simulink model "Electrical_System_2018b_obfs"  (R2019b)
settings: Solver=VariableStepAuto  StartTime=0.0  StopTime=5  RelTol=1e-3  AbsTol=1e-3  EnableMultiTasking=on
InitFcn:
  | Steady_State_Initialisation;
StopFcn:
  | %sscexplore(simlog);
  | %Logging
undefined symbols (not defined in the file): abrlhklxvp, aexgmhuedq, afmfmjnutg, afpphrjpnc, ahuxbyvruc, alarvljztt, amxnyqmnuw, aodrlwvqie, aolhmuplyq, aqpmguuqkg, auesgwirzl, aurophlnng, awamelrhru, ayfhvxflxn, azxkacuhqc, babszerikg, bawhdqanwq, bevoqecvei, bltjvqbchx, bmqsuewujl, bsmyqjfgnf, btvjbsmnve, bywgxqeadw, bziaduxaer, bzmcmdqocb, bzsvyvetat, ccsjnrbsih, cdvenygxwh, cedkrnslhx, cjheorclzs, cjrdshrtqx, ckhavyhcza, ckxewznhlz, cmrcgyiplk, conenicnws, cqkejbgjnn, csfnuwymhe, cunupkhwbh, cwzfvzuxxh, dcadmadufn, dcfponivnv, ddtrqjrhjn, dfhoxvkqas, dfrhtcwpne, dfvomcagjv, djijwylxea, dnmeqksrrm, dnzewbdkaa, dsqcykyxav, dtswwlttmm, ecumpidjtv, edegaywrct, ejjjsmnejc, eknqnehjdz, emvdetzouf, esxbqkbahr, etnkkbreiq, eunoiiiirw, ewewcuedir, fatkfxdhtc ... (+386)
libraries: fl_lib x802, ee_lib x362, fl_ps_legacy_lib x160, nesl_utility x85
(part 20 of 26)

== system Electrical_System_2018b_obfs/Redacted_1221/Redacted_7996/Redacted_7418/Redacted_4377/Redacted_6082/Redacted_6620 ==
  Redacted_2014 : ee_lib/Semiconductors & Converters/Diode  ModelType=gqiqleufpp  Vf=rciegaahyr V  Ron=izpyebfwtu Ohm  Goff=knahxehrum S  prmExp=gfxklcgmfk  I12=sbznuevzft A  V12=qpwzodqtgo V  IS=ebxfpmarae A  ec=cwkebwdiwj  I1=hqlohoyszw A  V1=mibkackcep V  RS=jhziukqmxk Ohm  Tmeas=tipcupyvvg degC  N_series=agpfoieknu  N_parallel=pauhaoalka  Rz=zxlwwxndwh Ohm  BV=swupfoviat V  C_param=ttoktqetan  CJ=mfxdwlmbvb pF  CJ0=ffeyzckaxr pF  VJ=nuecpjtket V  Mgrad=zfikmwifnf  Vvec=phbjpfbebd V  Cvec=jhnyxymlxo pF  FC=qfmmxpjbpo  Q_param=tjqqjjtelq  iRM=zutwrbrukx A  iF=pfiaynnkdw A  didt=zeupzzuvaz A/us  trr_factor=xhypptopno  trr=jkwajzgcje ns  Qrr=wowpcqfxws s*uA  TT=ypsxdlnldi ns  tau=nitvzeaztq ns  T_param=swaejwrfsv  IS_T2=xjhdogbuoa A  I1_T2=ldlggurlak A  V1_T2=obdohodlqe V  Tmeas2=tbryjoyfon degC  EG_param=erphnnwltu  EG=brjowwryvb eV  XTI_param=owdxpyfvwu  XTI=hgcqikgdha  dBVdT=lrzjaamqpw V/K  Tdevice=tcrbomkdjd degC  i_specify=off  i_priority=None  i=hqtjudspyd A  i_nominal_specify=off  i_nominal_unit=A  i_nominal_value=bwqxfkinvz  v_specify=off  v_priority=None  v=hjzmmprpyc V  v_nominal_specify=off  v_nominal_unit=V  v_nominal_value=njncclngsw  i_capacitor_specify=off  i_capacitor_priority=None  i_capacitor=ciyrjytfew A  i_capacitor_nominal_specify=off  i_capacitor_nominal_unit=A  i_capacitor_nominal_value=siexlgmunl  v_capacitor_specify=off  v_capacitor_priority=None  v_capacitor=xpshqsgilj V  v_capacitor_nominal_specify=off  v_capacitor_nominal_unit=V  v_capacitor_nominal_value=hpsiplsygj  power_dissipated_specify=off  power_dissipated_priority=None  power_dissipated=juqfttnpie W  power_dissipated_nominal_specify=off  power_dissipated_nominal_unit=W  power_dissipated_nominal_value=lyxbmpxuee  thermal_network_parameterization=ysuejmoxwn  Rth=finvmqpapu K/W  Rth_Foster=qosqwhtwdn K/W  thermal_mass_parameterization=swzmoavdkp  thermal_mass=ywjpsxqlmn J/K  thermal_mass_Foster=zzqhnpotok J/K  thermal_time_constant=ifknfrcsyy s  thermal_time_constant_Foster=pykgbenxxp s  thermal_mass_initial_temperatures=kgoranomvt degC
      settings: SourceProductName=Simscape Electrical  InternalSimscapePortConfiguration="{\"Bottom\":[],\"Left\":[{\"id\":\"p\",\"label\":\"\",\"type\":\"foundation.electrical.electrical\"},{\"id\":\"H\",\"label\":\"H\",\"type\":\"foundation.thermal.thermal\"}],\"Right\":[{\"id\":\"n\",\"label\":\"\",\"type\":\"foundation.electrical.electrical\"}],\"Top\":[]}"
  Redacted_2373 : fl_lib/Electrical/Electrical Elements/Switch  R_closed=kdyjcggfxg Ohm  G_open=afvdermyno 1/Ohm  Threshold=tjabhhlnxp  i_specify=off  i_priority=None  i=qurnjndsab A  i_nominal_specify=off  i_nominal_unit=A  i_nominal_value=znixxagswj  v_specify=off  v_priority=None  v=xqjhhmdgoi V  v_nominal_specify=off  v_nominal_unit=V  v_nominal_value=bwgubpgymn
      settings: SourceProductName=Simscape
  Redacted_328 : ee_lib/Passive/Thermal/Thermal Resistor  R=kxydmktclb K/W  T_specify=off  T_priority=None  T=vxwjbstjgr K  T_nominal_specify=off  T_nominal_unit=K  T_nominal_value=seidpjimmz  Q_specify=off  Q_priority=None  Q=ywgtndhhrq W  Q_nominal_specify=off  Q_nominal_unit=W  Q_nominal_value=kiultrtaba
      settings: SourceProductName=Simscape Electrical  SourceProductBaseCode=PS  InternalSimscapePortConfiguration="{\"Bottom\":[],\"Left\":[{\"id\":\"A\",\"label\":\"A\",\"type\":\"foundation.thermal.thermal\"}],\"Right\":[{\"id\":\"B\",\"label\":\"B\",\"type\":\"foundation.thermal.thermal\"}],\"Top\":[]}"
  Redacted_5690 : ee_lib/Passive/Thermal/Thermal Resistor  R=jddwcmhgli K/W  T_specify=off  T_priority=None  T=zezvrnfoms K  T_nominal_specify=off  T_nominal_unit=K  T_nominal_value=mzautmapaq  Q_specify=off  Q_priority=None  Q=yyadonrfbk W  Q_nominal_specify=off  Q_nominal_unit=W  Q_nominal_value=uclyfxddyt
      settings: SourceProductName=Simscape Electrical  SourceProductBaseCode=PS  InternalSimscapePortConfiguration="{\"Bottom\":[],\"Left\":[{\"id\":\"A\",\"label\":\"A\",\"type\":\"foundation.thermal.thermal\"}],\"Right\":[{\"id\":\"B\",\"label\":\"B\",\"type\":\"foundation.thermal.thermal\"}],\"Top\":[]}"
  Redacted_5845 : fl_lib/Electrical/Electrical Elements/Switch  R_closed=icjvxdmcka Ohm  G_open=kexskzpskw 1/Ohm  Threshold=ckhavyhcza  i_specify=off  i_priority=None  i=ahqiwrglzv A  i_nominal_specify=off  i_nominal_unit=A  i_nominal_value=mqjcwkekap  v_specify=off  v_priority=None  v=nvxykueeox V  v_nominal_specify=off  v_nominal_unit=V  v_nominal_value=ndecikrhmu
      settings: SourceProductName=Simscape
  Redacted_7283 : ee_lib/Semiconductors & Converters/Diode  ModelType=rzispxqwda  Vf=gnrpcrdaiq V  Ron=ghfqfgqnjp Ohm  Goff=ymfjoafqzi S  prmExp=tqesvxwkea  I12=gozxalvtjw A  V12=pfyubiyuoh V  IS=mbclrzefme A  ec=okvrwbwosn  I1=jpahbfupht A  V1=vpjuinocqb V  RS=brkyhzgmwm Ohm  Tmeas=zpdstripvt degC  N_series=stuuhiyehn  N_parallel=trqngxgybj  Rz=nzotohhllu Ohm  BV=opywdvhnir V  C_param=yuoevnzdrc  CJ=dhacxrqtkw pF  CJ0=mcyeruteos pF  VJ=mcmizpovly V  Mgrad=vsutktjlwr  Vvec=xuzjzmvewr V  Cvec=chlneajmrc pF  FC=nlhhtnylay  Q_param=cehpwvemhb  iRM=rlczpfgyem A  iF=ksurhnqwmp A  didt=idojsdbupn A/us  trr_factor=vejvrsmbmm  trr=kgmamwjxvx ns  Qrr=sefksjtwpk s*uA  TT=ifvfcwpbar ns  tau=mktlcufgsp ns  T_param=oprpphkwsn  IS_T2=ojtnhwzapa A  I1_T2=otxdgcfkfq A  V1_T2=fvsufutiqn V  Tmeas2=wipgwptrgf degC  EG_param=jbkevzjnlz  EG=ygoaixicyx eV  XTI_param=lgjkmxsxep  XTI=quhynflpcu  dBVdT=zwfbrmsbta V/K  Tdevice=phqcsvszoj degC  i_specify=off  i_priority=None  i=gjjcexnudv A  i_nominal_specify=off  i_nominal_unit=A  i_nominal_value=cfpddevnes  v_specify=off  v_priority=None  v=euxehncunu V  v_nominal_specify=off  v_nominal_unit=V  v_nominal_value=lplxzeyrex  i_capacitor_specify=off  i_capacitor_priority=None  i_capacitor=tbylysbvet A  i_capacitor_nominal_specify=off  i_capacitor_nominal_unit=A  i_capacitor_nominal_value=klnsswlrcx  v_capacitor_specify=off  v_capacitor_priority=None  v_capacitor=sxnwccbswb V  v_capacitor_nominal_specify=off  v_capacitor_nominal_unit=V  v_capacitor_nominal_value=yowydohudj  power_dissipated_specify=off  power_dissipated_priority=None  power_dissipated=cgphorjmje W  power_dissipated_nominal_specify=off  power_dissipated_nominal_unit=W  power_dissipated_nominal_value=fvywpxahim  thermal_network_parameterization=tyffilnlux  Rth=skkjpribxf K/W  Rth_Foster=hnqwerdzfk K/W  thermal_mass_parameterization=vwchogqojn  thermal_mass=xrttmmxuwx J/K  thermal_mass_Foster=oxwxslpupn J/K  thermal_time_constant=mxcjwvzono s  thermal_time_constant_Foster=gwwbtvmuug s  thermal_mass_initial_temperatures=claqdpboor degC
      settings: SourceProductName=Simscape Electrical  InternalSimscapePortConfiguration="{\"Bottom\":[],\"Left\":[{\"id\":\"p\",\"label\":\"\",\"type\":\"foundation.electrical.electrical\"},{\"id\":\"H\",\"label\":\"H\",\"type\":\"foundation.thermal.thermal\"}],\"Right\":[{\"id\":\"n\",\"label\":\"\",\"type\":\"foundation.electrical.electrical\"}],\"Top\":[]}"
  Redacted_9450 : ee_lib/Passive/Thermal/Thermal Resistor  R=wlxdrklwxe K/W  T_specify=off  T_priority=None  T=ncdbkbrldr K  T_nominal_specify=off  T_nominal_unit=K  T_nominal_value=tpldjyjupo  Q_specify=off  Q_priority=None  Q=wtqakfmuxk W  Q_nominal_specify=off  Q_nominal_unit=W  Q_nominal_value=wvihfdufoh
      settings: SourceProductName=Simscape Electrical  SourceProductBaseCode=PS  InternalSimscapePortConfiguration="{\"Bottom\":[],\"Left\":[{\"id\":\"A\",\"label\":\"A\",\"type\":\"foundation.thermal.thermal\"}],\"Right\":[{\"id\":\"B\",\"label\":\"B\",\"type\":\"foundation.thermal.thermal\"}],\"Top\":[]}"
  Redacted_4655 : PMIOPort  Side=Left
  Redacted_6502 : PMIOPort  Port=2  Side=Left
  Redacted_6154 : PMIOPort  Port=3  Side=Right
  Redacted_874 : PMIOPort  Port=4  Side=Right
  Redacted_3696 : PMIOPort  Port=5  Side=Left
  Redacted_2870 : PMIOPort  Port=6  Side=Right
  connections:
  Redacted_7283/LConn1 -- Redacted_6502/RConn1
  Redacted_7283/RConn1 -- Redacted_5845/LConn1
  Redacted_2014/LConn2 -- Redacted_9450/LConn1
  Redacted_6154/RConn1 -- Redacted_2373/RConn2
  Redacted_2014/LConn1 -- Redacted_2373/LConn1
  Redacted_4655/RConn1 -- Redacted_2014/RConn1
  Redacted_5690/RConn1 -- Redacted_328/LConn1 -- Redacted_9450/RConn1
  Redacted_2870/RConn1 -- Redacted_5845/RConn1 -- Redacted_2373/RConn1
  Redacted_874/RConn1 -- Redacted_5845/RConn2
  Redacted_328/RConn1 -- Redacted_3696/RConn1
  Redacted_7283/LConn2 -- Redacted_5690/LConn1

== system Electrical_System_2018b_obfs/Redacted_1221/Redacted_7996/Redacted_7418/Redacted_4377/Redacted_6082/Redacted_6805 ==
  Redacted_3337 : fl_lib/Electrical/Electrical Elements/Switch  R_closed=yxjpulldun Ohm  G_open=kegtkujuqm 1/Ohm  Threshold=liaknalfrc  i_specify=off  i_priority=None  i=vfyyawjcai A  i_nominal_specify=off  i_nominal_unit=A  i_nominal_value=qcjaunzuqi  v_specify=off  v_priority=None  v=swbfgzjayv V  v_nominal_specify=off  v_nominal_unit=V  v_nominal_value=ccklftegqq
      settings: SourceProductName=Simscape
  Redacted_4658 : ee_lib/Passive/Thermal/Thermal Resistor  R=cjheorclzs K/W  T_specify=off  T_priority=None  T=oxllrndvxl K  T_nominal_specify=off  T_nominal_unit=K  T_nominal_value=vttfcznyjj  Q_specify=off  Q_priority=None  Q=veltrvmbzh W  Q_nominal_specify=off  Q_nominal_unit=W  Q_nominal_value=iyxxiklgjl
      settings: SourceProductName=Simscape Electrical  SourceProductBaseCode=PS  InternalSimscapePortConfiguration="{\"Bottom\":[],\"Left\":[{\"id\":\"A\",\"label\":\"A\",\"type\":\"foundation.thermal.thermal\"}],\"Right\":[{\"id\":\"B\",\"label\":\"B\",\"type\":\"foundation.thermal.thermal\"}],\"Top\":[]}"
  Redacted_4994 : ee_lib/Passive/Thermal/Thermal Resistor  R=gypqteikkp K/W  T_specify=off  T_priority=None  T=oshyvpbftq K  T_nominal_specify=off  T_nominal_unit=K  T_nominal_value=ncwvhuakjs  Q_specify=off  Q_priority=None  Q=vojlmgegxo W  Q_nominal_specify=off  Q_nominal_unit=W  Q_nominal_value=fvyiuwsylh
      settings: SourceProductName=Simscape Electrical  SourceProductBaseCode=PS  InternalSimscapePortConfiguration="{\"Bottom\":[],\"Left\":[{\"id\":\"A\",\"label\":\"A\",\"type\":\"foundation.thermal.thermal\"}],\"Right\":[{\"id\":\"B\",\"label\":\"B\",\"type\":\"foundation.thermal.thermal\"}],\"Top\":[]}"
  Redacted_585 : fl_lib/Electrical/Electrical Elements/Switch  R_closed=wdigxdpfas Ohm  G_open=lafhprgygd 1/Ohm  Threshold=aolhmuplyq  i_specify=off  i_priority=None  i=vcdeejycwc A  i_nominal_specify=off  i_nominal_unit=A  i_nominal_value=ershxznodz  v_specify=off  v_priority=None  v=irimjohetc V  v_nominal_specify=off  v_nominal_unit=V  v_nominal_value=bejlrppchs
      settings: SourceProductName=Simscape
  Redacted_7139 : ee_lib/Passive/Thermal/Thermal Resistor  R=qokdevsgjk K/W  T_specify=off  T_priority=None  T=zzfqycdapp K  T_nominal_specify=off  T_nominal_unit=K  T_nominal_value=mlevfhnhhd  Q_specify=off  Q_priority=None  Q=grrzcklvos W  Q_nominal_specify=off  Q_nominal_unit=W  Q_nominal_value=pjoujutyxi
      settings: SourceProductName=Simscape Electrical  SourceProductBaseCode=PS  InternalSimscapePortConfiguration="{\"Bottom\":[],\"Left\":[{\"id\":\"A\",\"label\":\"A\",\"type\":\"foundation.thermal.thermal\"}],\"Right\":[{\"id\":\"B\",\"label\":\"B\",\"type\":\"foundation.thermal.thermal\"}],\"Top\":[]}"
  Redacted_7477 : ee_lib/Semiconductors & Converters/Diode  ModelType=siopqsdkke  Vf=vlytbuckhg V  Ron=dnkirfiwtb Ohm  Goff=hybfzeduao S  prmExp=kwsebrwvgd  I12=kfsmyoqzna A  V12=hnkonhxsbr V  IS=isykihjzmv A  ec=yrzkujitpm  I1=dhfqeyhuyd A  V1=zgsewcozym V  RS=mpcljitwmr Ohm  Tmeas=ebrkobcskh degC  N_series=cblbppjhmu  N_parallel=gcijoxluxf  Rz=wwudmfsgii Ohm  BV=ywubfrqvzl V  C_param=ufueahyemx  CJ=ucffunbhjr pF  CJ0=gvgqkuhnif pF  VJ=eafaphsqye V  Mgrad=stbyrblvuf  Vvec=lqtyuphlxe V  Cvec=kwepiurgav pF  FC=bocziebzeh  Q_param=axqhxumszd  iRM=mvlaklwalt A  iF=fvdwflwmxq A  didt=yduxgmzydl A/us  trr_factor=xzyzzmdibz  trr=mqeokcuxni ns  Qrr=eacuvomyfz s*uA  TT=wqeovxwgoy ns  tau=icgjzejdcm ns  T_param=qvfyrqpkio  IS_T2=tyrvatdotb A  I1_T2=hdybxwnxgg A  V1_T2=ocskkzbdfs V  Tmeas2=roeazaidao degC  EG_param=ltrdisotaf  EG=irbxnhvhnf eV  XTI_param=uvozxekhry  XTI=vcneuywdti  dBVdT=bjxifjvwqu V/K  Tdevice=lzvjtpnwvt degC  i_specify=off  i_priority=None  i=yyxgeutxkj A  i_nominal_specify=off  i_nominal_unit=A  i_nominal_value=hkglitcqqq  v_specify=off  v_priority=None  v=ncxmzzrzjk V  v_nominal_specify=off  v_nominal_unit=V  v_nominal_value=lsdkgzvlcc  i_capacitor_specify=off  i_capacitor_priority=None  i_capacitor=xlhxuygwjg A  i_capacitor_nominal_specify=off  i_capacitor_nominal_unit=A  i_capacitor_nominal_value=drafximium  v_capacitor_specify=off  v_capacitor_priority=None  v_capacitor=jpwbpwcwee V  v_capacitor_nominal_specify=off  v_capacitor_nominal_unit=V  v_capacitor_nominal_value=hdkefavzlf  power_dissipated_specify=off  power_dissipated_priority=None  power_dissipated=sarhttkwql W  power_dissipated_nominal_specify=off  power_dissipated_nominal_unit=W  power_dissipated_nominal_value=mavrwpomwo  thermal_network_parameterization=lrcygnfvyi  Rth=srgsdzcvpf K/W  Rth_Foster=twreyxnsjr K/W  thermal_mass_parameterization=nbdhbesxpg  thermal_mass=rxfluekgwa J/K  thermal_mass_Foster=cklbgtlgis J/K  thermal_time_constant=lubwmajmlm s  thermal_time_constant_Foster=tnksfxwvyl s  thermal_mass_initial_temperatures=cgflfnvnmx degC
      settings: SourceProductName=Simscape Electrical  InternalSimscapePortConfiguration="{\"Bottom\":[],\"Left\":[{\"id\":\"p\",\"label\":\"\",\"type\":\"foundation.electrical.electrical\"},{\"id\":\"H\",\"label\":\"H\",\"type\":\"foundation.thermal.thermal\"}],\"Right\":[{\"id\":\"n\",\"label\":\"\",\"type\":\"foundation.electrical.electrical\"}],\"Top\":[]}"
  Redacted_7606 : ee_lib/Semiconductors & Converters/Diode  ModelType=uzkzrdmcdd  Vf=rmmzroxgij V  Ron=gmhtedufnv Ohm  Goff=jjlyzatkvo S  prmExp=veirngjlfx  I12=qvvduldzrp A  V12=zynirzrnpf V  IS=wxxxvpohgl A  ec=fplwtkcwyr  I1=kpelximtdu A  V1=wylxnblunc V  RS=jbawbkggmq Ohm  Tmeas=bayoigkdqj degC  N_series=bgulwrfglp  N_parallel=khxpeniani  Rz=lylxbzffke Ohm  BV=csvlicgnxf V  C_param=wxpimfnkor  CJ=rlhvodbzhe pF  CJ0=tjvrgdxdbq pF  VJ=kymohesfqq V  Mgrad=exkywwsvhl  Vvec=xkmmhtmqkw V  Cvec=fymvnufolq pF  FC=tgeertiozj  Q_param=yijflpurri  iRM=fjtqudaeyk A  iF=opauyjbtnw A  didt=wdwvlihuzw A/us  trr_factor=olttdrnnql  trr=egrhxizosf ns  Qrr=lsshsmphht s*uA  TT=edtwkkrcoh ns  tau=raidgjkdvk ns  T_param=ahbhdfhjai  IS_T2=ekcwzeqyaw A  I1_T2=orjhprekra A  V1_T2=ztliozxhxg V  Tmeas2=tfrmoaghps degC  EG_param=oapwdsvvtf  EG=irybcfpwlp eV  XTI_param=olnutyjuem  XTI=xesgdyozdg  dBVdT=oepeppyrik V/K  Tdevice=jpqttphnsz degC  i_specify=off  i_priority=None  i=svdtmokjoo A  i_nominal_specify=off  i_nominal_unit=A  i_nominal_value=abngkcnppn  v_specify=off  v_priority=None  v=uaenfqikhz V  v_nominal_specify=off  v_nominal_unit=V  v_nominal_value=ptrurkjdbb  i_capacitor_specify=off  i_capacitor_priority=None  i_capacitor=qrsrlqghol A  i_capacitor_nominal_specify=off  i_capacitor_nominal_unit=A  i_capacitor_nominal_value=ndtskdbzxd  v_capacitor_specify=off  v_capacitor_priority=None  v_capacitor=drqgaqzvul V  v_capacitor_nominal_specify=off  v_capacitor_nominal_unit=V  v_capacitor_nominal_value=ufwludarpz  power_dissipated_specify=off  power_dissipated_priority=None  power_dissipated=zarwoastjt W  power_dissipated_nominal_specify=off  power_dissipated_nominal_unit=W  power_dissipated_nominal_value=yqmounopok  thermal_network_parameterization=lbqkpegruw  Rth=wfrzaaeyrf K/W  Rth_Foster=orzhpmmvoh K/W  thermal_mass_parameterization=cvfxrzqybx  thermal_mass=vploeluiax J/K  thermal_mass_Foster=fxfiinqkbf J/K  thermal_time_constant=wfhctbbpau s  thermal_time_constant_Foster=nxdwubasmi s  thermal_mass_initial_temperatures=izxzueqzis degC
      settings: SourceProductName=Simscape Electrical  InternalSimscapePortConfiguration="{\"Bottom\":[],\"Left\":[{\"id\":\"p\",\"label\":\"\",\"type\":\"foundation.electrical.electrical\"},{\"id\":\"H\",\"label\":\"H\",\"type\":\"foundation.thermal.thermal\"}],\"Right\":[{\"id\":\"n\",\"label\":\"\",\"type\":\"foundation.electrical.electrical\"}],\"Top\":[]}"
  Redacted_2990 : PMIOPort  Side=Left
  Redacted_5799 : PMIOPort  Port=2  Side=Left
  Redacted_5060 : PMIOPort  Port=3  Side=Right
  Redacted_1541 : PMIOPort  Port=4  Side=Right
  Redacted_1201 : PMIOPort  Port=5  Side=Left
  Redacted_6993 : PMIOPort  Port=6  Side=Right
  connections:
  Redacted_7477/LConn1 -- Redacted_5799/RConn1
  Redacted_7477/RConn1 -- Redacted_3337/LConn1
  Redacted_7606/LConn2 -- Redacted_7139/LConn1
  Redacted_5060/RConn1 -- Redacted_585/RConn2
  Redacted_7606/LConn1 -- Redacted_585/LConn1
  Redacted_2990/RConn1 -- Redacted_7606/RConn1
  Redacted_4994/RConn1 -- Redacted_4658/LConn1 -- Redacted_7139/RConn1
  Redacted_6993/RConn1 -- Redacted_3337/RConn1 -- Redacted_585/RConn1
  Redacted_1541/RConn1 -- Redacted_3337/RConn2
  Redacted_4658/RConn1 -- Redacted_1201/RConn1
  Redacted_7477/LConn2 -- Redacted_4994/LConn1

== system Electrical_System_2018b_obfs/Redacted_1221/Redacted_7996/Redacted_7418/Redacted_4377/Redacted_6082/Redacted_7051 ==
  Neutral_Negative : Subsystem  VariantControl=Variant1
  Positive_Neutral : Subsystem  VariantControl=Variant3
  Redacted_1021 : Subsystem  VariantControl=Variant2
  Redacted_2697 : PMIOPort  Side=Left
  Redacted_1518 : PMIOPort  Port=2  Side=Left
  Redacted_2395 : PMIOPort  Port=3  Side=Left
  Redacted_3537 : PMIOPort  Port=4  Side=Right
  Redacted_8383 : PMIOPort  Port=5  Side=Right

== system Electrical_System_2018b_obfs/Redacted_1221/Redacted_7996/Redacted_7418/Redacted_4377/Redacted_6082/Redacted_7167 ==
  Redacted_1303 : ee_lib/Passive/Thermal/Thermal Resistor  R=zbwmizebwe K/W  T_specify=off  T_priority=None  T=rqecdygusj K  T_nominal_specify=off  T_nominal_unit=K  T_nominal_value=lamojxsfir  Q_specify=off  Q_priority=None  Q=dlcstliuma W  Q_nominal_specify=off  Q_nominal_unit=W  Q_nominal_value=tijbovpdks
      settings: SourceProductName=Simscape Electrical  SourceProductBaseCode=PS  InternalSimscapePortConfiguration="{\"Bottom\":[],\"Left\":[{\"id\":\"A\",\"label\":\"A\",\"type\":\"foundation.thermal.thermal\"}],\"Right\":[{\"id\":\"B\",\"label\":\"B\",\"type\":\"foundation.thermal.thermal\"}],\"Top\":[]}"
  Redacted_2941 : ee_lib/Passive/Thermal/Thermal Resistor  R=dfhoxvkqas K/W  T_specify=off  T_priority=None  T=jlvbuiuarv K  T_nominal_specify=off  T_nominal_unit=K  T_nominal_value=nfbcsilcng  Q_specify=off  Q_priority=None  Q=dpepytyjnn W  Q_nominal_specify=off  Q_nominal_unit=W  Q_nominal_value=eutxhekizl
      settings: SourceProductName=Simscape Electrical  SourceProductBaseCode=PS  InternalSimscapePortConfiguration="{\"Bottom\":[],\"Left\":[{\"id\":\"A\",\"label\":\"A\",\"type\":\"foundation.thermal.thermal\"}],\"Right\":[{\"id\":\"B\",\"label\":\"B\",\"type\":\"foundation.thermal.thermal\"}],\"Top\":[]}"
  Redacted_3917 : fl_lib/Electrical/Electrical Elements/Switch  R_closed=eomshdfjtq Ohm  G_open=eawwctyuef 1/Ohm  Threshold=nqsqjnzstw  i_specify=off  i_priority=None  i=gvnqmmhjic A  i_nominal_specify=off  i_nominal_unit=A  i_nominal_value=mwmoxwopsr  v_specify=off  v_priority=None  v=gqkvmmaeai V  v_nominal_specify=off  v_nominal_unit=V  v_nominal_value=euweqcpati
      settings: SourceProductName=Simscape
  Redacted_615 : ee_lib/Semiconductors & Converters/Diode  ModelType=pgkejxjdjs  Vf=xdcykktqir V  Ron=eayqiytylj Ohm  Goff=xzfhydetzu S  prmExp=tdufjhjcbn  I12=hparrpdjbc A  V12=zqwdfgidjk V  IS=pexhzonywb A  ec=mqktskfdqf  I1=tcyogdxzfi A  V1=baszszoezq V  RS=bxlpeeaqsl Ohm  Tmeas=tbiklxcmxf degC  N_series=eikuqooelh  N_parallel=xnclysjpwz  Rz=svpfhmlvnd Ohm  BV=ymvvdallkk V  C_param=auiedyngha  CJ=tdcyeazvtn pF  CJ0=yhsttyriji pF  VJ=oyfcsuwtca V  Mgrad=ssglilauuc  Vvec=tcaqzincyj V  Cvec=gaeocfhldf pF  FC=govhvunkzb  Q_param=gwouayihiu  iRM=gmuyhfsqfq A  iF=qgolhenzzh A  didt=roskpmqafp A/us  trr_factor=rgtcsetsdw  trr=evtippvdri ns  Qrr=asluyjhcqx s*uA  TT=hthltjmqxb ns  tau=mpvzluyvkf ns  T_param=ffjfzvgxwk  IS_T2=wfxjsgcogp A  I1_T2=lfwejdvrcx A  V1_T2=peppezqval V  Tmeas2=yreqhveqgb degC  EG_param=dqtocyjvqe  EG=aodkzgenxb eV  XTI_param=ncbiefewza  XTI=uvmuxgsyie  dBVdT=ejtxbvomre V/K  Tdevice=gpojnnavgh degC  i_specify=off  i_priority=None  i=ylnqkojcnb A  i_nominal_specify=off  i_nominal_unit=A  i_nominal_value=rmjbnjurkm  v_specify=off  v_priority=None  v=igzgyorjhh V  v_nominal_specify=off  v_nominal_unit=V  v_nominal_value=llpsdzaxev  i_capacitor_specify=off  i_capacitor_priority=None  i_capacitor=phioximztf A  i_capacitor_nominal_specify=off  i_capacitor_nominal_unit=A  i_capacitor_nominal_value=zpfkwwvufw  v_capacitor_specify=off  v_capacitor_priority=None  v_capacitor=orgrxnzlgw V  v_capacitor_nominal_specify=off  v_capacitor_nominal_unit=V  v_capacitor_nominal_value=kmrqvqymze  power_dissipated_specify=off  power_dissipated_priority=None  power_dissipated=tckulawdha W  power_dissipated_nominal_specify=off  power_dissipated_nominal_unit=W  power_dissipated_nominal_value=zqxclxuaeb  thermal_network_parameterization=xbiounqwbn  Rth=cthaouvkmz K/W  Rth_Foster=ujuovdsbwu K/W  thermal_mass_parameterization=yndypypslu  thermal_mass=yqwtrsfarw J/K  thermal_mass_Foster=uknzmftfxw J/K  thermal_time_constant=gadiboyzjf s  thermal_time_constant_Foster=oonjgnxbhv s  thermal_mass_initial_temperatures=dwinptcuvn degC
      settings: SourceProductName=Simscape Electrical  InternalSimscapePortConfiguration="{\"Bottom\":[],\"Left\":[{\"id\":\"p\",\"label\":\"\",\"type\":\"foundation.electrical.electrical\"},{\"id\":\"H\",\"label\":\"H\",\"type\":\"foundation.thermal.thermal\"}],\"Right\":[{\"id\":\"n\",\"label\":\"\",\"type\":\"foundation.electrical.electrical\"}],\"Top\":[]}"
  Redacted_6479 : fl_lib/Electrical/Electrical Elements/Switch  R_closed=pbrfqnpyma Ohm  G_open=cpoeuurqry 1/Ohm  Threshold=xzfpsnkrcq  i_specify=off  i_priority=None  i=svmhsuqoiq A  i_nominal_specify=off  i_nominal_unit=A  i_nominal_value=grkinioqrq  v_specify=off  v_priority=None  v=bfmdrrxebu V  v_nominal_specify=off  v_nominal_unit=V  v_nominal_value=tuetnympor
      settings: SourceProductName=Simscape
  Redacted_6758 : ee_lib/Passive/Thermal/Thermal Resistor  R=udvbnpfogk K/W  T_specify=off  T_priority=None  T=stamifxejg K  T_nominal_specify=off  T_nominal_unit=K  T_nominal_value=jpdxtgtapc  Q_specify=off  Q_priority=None  Q=ijcjukjuex W  Q_nominal_specify=off  Q_nominal_unit=W  Q_nominal_value=ruzflvabxw
      settings: SourceProductName=Simscape Electrical  SourceProductBaseCode=PS  InternalSimscapePortConfiguration="{\"Bottom\":[],\"Left\":[{\"id\":\"A\",\"label\":\"A\",\"type\":\"foundation.thermal.thermal\"}],\"Right\":[{\"id\":\"B\",\"label\":\"B\",\"type\":\"foundation.thermal.thermal\"}],\"Top\":[]}"
  Redacted_950 : ee_lib/Semiconductors & Converters/Diode  ModelType=jinkuwtpek  Vf=atuwmhjlss V  Ron=nznnxbdyxy Ohm  Goff=ihbvkszwml S  prmExp=mibtplliji  I12=iyuliuqmcx A  V12=klduiyaqij V  IS=ikslmrckpw A  ec=zngamoehie  I1=jmqjtcgqqy A  V1=qeujplmsly V  RS=prjefekpfj Ohm  Tmeas=xbblauhoxo degC  N_series=zriukxbglf  N_parallel=xywdgylyct  Rz=mlyrjcrutc Ohm  BV=azpesxbvkt V  C_param=iwaqnxrihq  CJ=efrhdiawni pF  CJ0=wggafursrp pF  VJ=kimodzupzz V  Mgrad=zqomfqqbkp  Vvec=nmespqdqtf V  Cvec=ptwbjcbecf pF  FC=rhpfuhhgyh  Q_param=irgquspdkp  iRM=juwqonlivh A  iF=ngzsvssqdj A  didt=qpzzvxqyny A/us  trr_factor=ytjldsqsba  trr=ynapedjysl ns  Qrr=cxbfwkibab s*uA  TT=qdlmrgrjbk ns  tau=gxbazwmswf ns  T_param=jeqpakxjhj  IS_T2=oyhthfujhz A  I1_T2=slwpnostwc A  V1_T2=ufjvlweifr V  Tmeas2=dmcyrgyzee degC  EG_param=txmgcwnshd  EG=awhwjuusqu eV  XTI_param=ciqcncwotj  XTI=sbuczetxrl  dBVdT=vvkuzgntho V/K  Tdevice=ayjozqrwzo degC  i_specify=off  i_priority=None  i=lfrhocvsab A  i_nominal_specify=off  i_nominal_unit=A  i_nominal_value=ltsgntbaxv  v_specify=off  v_priority=None  v=etlymrjkwh V  v_nominal_specify=off  v_nominal_unit=V  v_nominal_value=epreckwkhm  i_capacitor_specify=off  i_capacitor_priority=None  i_capacitor=tmlxdjnhjw A  i_capacitor_nominal_specify=off  i_capacitor_nominal_unit=A  i_capacitor_nominal_value=qqxajawsrd  v_capacitor_specify=off  v_capacitor_priority=None  v_capacitor=upkznbdmiq V  v_capacitor_nominal_specify=off  v_capacitor_nominal_unit=V  v_capacitor_nominal_value=dtybisinlb  power_dissipated_specify=off  power_dissipated_priority=None  power_dissipated=hsiyqtyqwk W  power_dissipated_nominal_specify=off  power_dissipated_nominal_unit=W  power_dissipated_nominal_value=warucurcbx  thermal_network_parameterization=fzipsrgnag  Rth=uxblvsvlml K/W  Rth_Foster=lcjkmpdgtw K/W  thermal_mass_parameterization=pcvahjrfam  thermal_mass=cugzbrnibs J/K  thermal_mass_Foster=sinoggzltj J/K  thermal_time_constant=afzkjcdnxg s  thermal_time_constant_Foster=ypnpugavcs s  thermal_mass_initial_temperatures=kinrukpyro degC
      settings: SourceProductName=Simscape Electrical  InternalSimscapePortConfiguration="{\"Bottom\":[],\"Left\":[{\"id\":\"p\",\"label\":\"\",\"type\":\"foundation.electrical.electrical\"},{\"id\":\"H\",\"label\":\"H\",\"type\":\"foundation.thermal.thermal\"}],\"Right\":[{\"id\":\"n\",\"label\":\"\",\"type\":\"foundation.electrical.electrical\"}],\"Top\":[]}"
  Redacted_4250 : PMIOPort  Side=Left
  Redacted_3366 : PMIOPort  Port=2  Side=Left
  Redacted_6205 : PMIOPort  Port=3  Side=Right
  Redacted_8107 : PMIOPort  Port=4  Side=Right
  Redacted_7175 : PMIOPort  Port=5  Side=Left
  Redacted_7678 : PMIOPort  Port=6  Side=Right
  connections:
  Redacted_615/LConn1 -- Redacted_3366/RConn1
  Redacted_615/RConn1 -- Redacted_6479/LConn1
  Redacted_950/LConn2 -- Redacted_2941/LConn1
  Redacted_6205/RConn1 -- Redacted_3917/RConn2
  Redacted_950/LConn1 -- Redacted_3917/LConn1
  Redacted_4250/RConn1 -- Redacted_950/RConn1
  Redacted_6758/RConn1 -- Redacted_1303/LConn1 -- Redacted_2941/RConn1
  Redacted_7678/RConn1 -- Redacted_6479/RConn1 -- Redacted_3917/RConn1
  Redacted_8107/RConn1 -- Redacted_6479/RConn2
  Redacted_1303/RConn1 -- Redacted_7175/RConn1
  Redacted_615/LConn2 -- Redacted_6758/LConn1

== system Electrical_System_2018b_obfs/Redacted_1221/Redacted_7996/Redacted_7418/Redacted_4377/Redacted_6082/Redacted_7871 ==
  Redacted_1150 : ee_lib/Passive/Thermal/Thermal Resistor  R=wnyhcrensu K/W  T_specify=off  T_priority=None  T=hfmwboisgl K  T_nominal_specify=off  T_nominal_unit=K  T_nominal_value=omfgbcxeiw  Q_specify=off  Q_priority=None  Q=jyeccfnuuv W  Q_nominal_specify=off  Q_nominal_unit=W  Q_nominal_value=kbomgljmud
      settings: SourceProductName=Simscape Electrical  SourceProductBaseCode=PS  InternalSimscapePortConfiguration="{\"Bottom\":[],\"Left\":[{\"id\":\"A\",\"label\":\"A\",\"type\":\"foundation.thermal.thermal\"}],\"Right\":[{\"id\":\"B\",\"label\":\"B\",\"type\":\"foundation.thermal.thermal\"}],\"Top\":[]}"
  Redacted_163 : fl_lib/Electrical/Electrical Elements/Switch  R_closed=wdukvpamow Ohm  G_open=xulqxrrjnv 1/Ohm  Threshold=qhmovogayg  i_specify=off  i_priority=None  i=uohgsyxugo A  i_nominal_specify=off  i_nominal_unit=A  i_nominal_value=woebaudwry  v_specify=off  v_priority=None  v=vemtymvmmi V  v_nominal_specify=off  v_nominal_unit=V  v_nominal_value=emvbxsbdsz
      settings: SourceProductName=Simscape
  Redacted_4906 : ee_lib/Semiconductors & Converters/Diode  ModelType=lisxnbujfq  Vf=xetfnwixtl V  Ron=kgggytotak Ohm  Goff=dicegnkmns S  prmExp=fsccnkszzi  I12=rkhncbyaxg A  V12=amfquhqfri V  IS=exemtgyddq A  ec=usfpzulpqi  I1=ugfovaezax A  V1=oljxivlmqp V  RS=dazrmfhoxo Ohm  Tmeas=baitckeesm degC  N_series=hfppshhhyr  N_parallel=rjxplrcndp  Rz=fabwipzqjc Ohm  BV=wyrpdjzqjf V  C_param=qgwqtktiiq  CJ=wbrnhtezpt pF  CJ0=phxqhonqpj pF  VJ=eteydoyhly V  Mgrad=glhtwvcvqy  Vvec=hwlxeyydpv V  Cvec=hxporvcfni pF  FC=gjviwqnvyt  Q_param=ncmzgihjzz  iRM=yvoogxejtg A  iF=qnmfqdbeto A  didt=agfovrodto A/us  trr_factor=frcqxuvvia  trr=hbqrwrvnxm ns  Qrr=fdoqfarsjb s*uA  TT=slfzkacqdx ns  tau=alaeanzbod ns  T_param=nuitneutsg  IS_T2=craloeoioz A  I1_T2=wjjsiamplw A  V1_T2=tewsfpvrmq V  Tmeas2=gxtdnafxpo degC  EG_param=wlioyiusag  EG=cpoejbuzyv eV  XTI_param=dddqpnqtzc  XTI=qrfykfwguz  dBVdT=ucurhhzfza V/K  Tdevice=rczcbfyedr degC  i_specify=off  i_priority=None  i=zzdxemwvng A  i_nominal_specify=off  i_nominal_unit=A  i_nominal_value=kfkirmacjn  v_specify=off  v_priority=None  v=uajyhxnboc V  v_nominal_specify=off  v_nominal_unit=V  v_nominal_value=jqepkydgfh  i_capacitor_specify=off  i_capacitor_priority=None  i_capacitor=rrmwbvgmcc A  i_capacitor_nominal_specify=off  i_capacitor_nominal_unit=A  i_capacitor_nominal_value=pjbytllgoo  v_capacitor_specify=off  v_capacitor_priority=None  v_capacitor=pfzlffxyis V  v_capacitor_nominal_specify=off  v_capacitor_nominal_unit=V  v_capacitor_nominal_value=rwblhtqxum  power_dissipated_specify=off  power_dissipated_priority=None  power_dissipated=ezbuvvjzbd W  power_dissipated_nominal_specify=off  power_dissipated_nominal_unit=W  power_dissipated_nominal_value=bhaqvsgfxr  thermal_network_parameterization=kyfbufrfys  Rth=rdswkjtiwa K/W  Rth_Foster=qshnyhfbmq K/W  thermal_mass_parameterization=gvhwjtzboo  thermal_mass=bdoomqzqok J/K  thermal_mass_Foster=anntstrfod J/K  thermal_time_constant=jfrqkttoqa s  thermal_time_constant_Foster=gslnrdmbpc s  thermal_mass_initial_temperatures=ucxtllsqhb degC
      settings: SourceProductName=Simscape Electrical  InternalSimscapePortConfiguration="{\"Bottom\":[],\"Left\":[{\"id\":\"p\",\"label\":\"\",\"type\":\"foundation.electrical.electrical\"},{\"id\":\"H\",\"label\":\"H\",\"type\":\"foundation.thermal.thermal\"}],\"Right\":[{\"id\":\"n\",\"label\":\"\",\"type\":\"foundation.electrical.electrical\"}],\"Top\":[]}"
  Redacted_5585 : fl_lib/Electrical/Electrical Elements/Switch  R_closed=gnrmopaexe Ohm  G_open=orsehmpisd 1/Ohm  Threshold=uztftemjgo  i_specify=off  i_priority=None  i=beydlfyovg A  i_nominal_specify=off  i_nominal_unit=A  i_nominal_value=iaidkfrlwq  v_specify=off  v_priority=None  v=zwfzhspjsy V  v_nominal_specify=off  v_nominal_unit=V  v_nominal_value=hnducacwcv
      settings: SourceProductName=Simscape
  Redacted_6192 : ee_lib/Semiconductors & Converters/Diode  ModelType=ptnynyqzgs  Vf=tkcshdmnfy V  Ron=etdxecgxkr Ohm  Goff=updvlgzhxi S  prmExp=bdmrzzzqpe  I12=sdcvfvczxq A  V12=qxwxvafkrp V  IS=fjehcmaddz A  ec=rcfxzuuzkz  I1=bbqivzbpbn A  V1=jbzephfaei V  RS=jfqjrslbtb Ohm  Tmeas=nmsknhwbdm degC  N_series=upbnprrhsm  N_parallel=gychkiuesj  Rz=ekjrkafpjm Ohm  BV=izllxqqtbw V  C_param=chrhwjdcia  CJ=zewhvymjzh pF  CJ0=xysumvzksz pF  VJ=plgvwexltq V  Mgrad=lfxmdopixh  Vvec=rhhplxfzfv V  Cvec=btxmrjnrpv pF  FC=gllfdejxcp  Q_param=jqpclwrtup  iRM=uzrdiaqfpb A  iF=zfvqwesedg A  didt=zxsbiuiqyg A/us  trr_factor=sbxmtvfbhj  trr=wpldszobql ns  Qrr=rgofeflbzu s*uA  TT=rydmpcnssa ns  tau=bhbpgrjiqy ns  T_param=utvpupdfuz  IS_T2=hbepvkcqcu A  I1_T2=gjnwhuwyhq A  V1_T2=iliyqurzbt V  Tmeas2=zejnxlzety degC  EG_param=cuajkktsgm  EG=goqdzkjwzg eV  XTI_param=pnvmcekqru  XTI=bkscbkgzda  dBVdT=mkrrrntnlw V/K  Tdevice=tkgdybdqcd degC  i_specify=off  i_priority=None  i=wgjngnbzpn A  i_nominal_specify=off  i_nominal_unit=A  i_nominal_value=ileaslxatl  v_specify=off  v_priority=None  v=agtzcmtlle V  v_nominal_specify=off  v_nominal_unit=V  v_nominal_value=vwqtyzlgqu  i_capacitor_specify=off  i_capacitor_priority=None  i_capacitor=eizgtbmzgc A  i_capacitor_nominal_specify=off  i_capacitor_nominal_unit=A  i_capacitor_nominal_value=vlhejuzknm  v_capacitor_specify=off  v_capacitor_priority=None  v_capacitor=sfnrfbvwbg V  v_capacitor_nominal_specify=off  v_capacitor_nominal_unit=V  v_capacitor_nominal_value=mnvorbtega  power_dissipated_specify=off  power_dissipated_priority=None  power_dissipated=terqltrajz W  power_dissipated_nominal_specify=off  power_dissipated_nominal_unit=W  power_dissipated_nominal_value=akhswoieim  thermal_network_parameterization=aqtnipjlzq  Rth=fvgepqsrwq K/W  Rth_Foster=wcabkcdyac K/W  thermal_mass_parameterization=baajrlnryr  thermal_mass=jkrfnomsau J/K  thermal_mass_Foster=bqnvprbfcb J/K  thermal_time_constant=mwpyhcvjxq s  thermal_time_constant_Foster=nxhccxykrw s  thermal_mass_initial_temperatures=dnnydknyte degC
      settings: SourceProductName=Simscape Electrical  InternalSimscapePortConfiguration="{\"Bottom\":[],\"Left\":[{\"id\":\"p\",\"label\":\"\",\"type\":\"foundation.electrical.electrical\"},{\"id\":\"H\",\"label\":\"H\",\"type\":\"foundation.thermal.thermal\"}],\"Right\":[{\"id\":\"n\",\"label\":\"\",\"type\":\"foundation.electrical.electrical\"}],\"Top\":[]}"
  Redacted_8694 : ee_lib/Passive/Thermal/Thermal Resistor  R=tvtoespfwy K/W  T_specify=off  T_priority=None  T=vzxlafqipt K  T_nominal_specify=off  T_nominal_unit=K  T_nominal_value=cbqqygtnvn  Q_specify=off  Q_priority=None  Q=szwiasewfs W  Q_nominal_specify=off  Q_nominal_unit=W  Q_nominal_value=bbrfndpujl
      settings: SourceProductName=Simscape Electrical  SourceProductBaseCode=PS  InternalSimscapePortConfiguration="{\"Bottom\":[],\"Left\":[{\"id\":\"A\",\"label\":\"A\",\"type\":\"foundation.thermal.thermal\"}],\"Right\":[{\"id\":\"B\",\"label\":\"B\",\"type\":\"foundation.thermal.thermal\"}],\"Top\":[]}"
  Redacted_9167 : ee_lib/Passive/Thermal/Thermal Resistor  R=cjrdshrtqx K/W  T_specify=off  T_priority=None  T=xdavxkvlqw K  T_nominal_specify=off  T_nominal_unit=K  T_nominal_value=bgekadzhxq  Q_specify=off  Q_priority=None  Q=jtdqtarogq W  Q_nominal_specify=off  Q_nominal_unit=W  Q_nominal_value=pabocztlon
      settings: SourceProductName=Simscape Electrical  SourceProductBaseCode=PS  InternalSimscapePortConfiguration="{\"Bottom\":[],\"Left\":[{\"id\":\"A\",\"label\":\"A\",\"type\":\"foundation.thermal.thermal\"}],\"Right\":[{\"id\":\"B\",\"label\":\"B\",\"type\":\"foundation.thermal.thermal\"}],\"Top\":[]}"
  Redacted_2241 : PMIOPort  Side=Left
  Redacted_3211 : PMIOPort  Port=2  Side=Left
  Redacted_9222 : PMIOPort  Port=3  Side=Right
  Redacted_2161 : PMIOPort  Port=4  Side=Right
  Redacted_7477 : PMIOPort  Port=5  Side=Left
  Redacted_8994 : PMIOPort  Port=6  Side=Right
  connections:
  Redacted_6192/LConn1 -- Redacted_3211/RConn1
  Redacted_6192/RConn1 -- Redacted_163/LConn1
  Redacted_4906/LConn2 -- Redacted_9167/LConn1
  Redacted_9222/RConn1 -- Redacted_5585/RConn2
  Redacted_4906/LConn1 -- Redacted_5585/LConn1
  Redacted_2241/RConn1 -- Redacted_4906/RConn1
  Redacted_8694/RConn1 -- Redacted_1150/LConn1 -- Redacted_9167/RConn1
  Redacted_8994/RConn1 -- Redacted_163/RConn1 -- Redacted_5585/RConn1
  Redacted_2161/RConn1 -- Redacted_163/RConn2
  Redacted_1150/RConn1 -- Redacted_7477/RConn1
  Redacted_6192/LConn2 -- Redacted_8694/LConn1

== system Electrical_System_2018b_obfs/Redacted_1221/Redacted_7996/Redacted_7418/Redacted_4377/Redacted_6082/Redacted_7884 ==
  Neutral_Negative : Subsystem  VariantControl=Variant1
  Positive_Neutral : Subsystem  VariantControl=Variant3
  Redacted_81 : Subsystem  VariantControl=Variant2
  Redacted_6224 : PMIOPort  Side=Left
  Redacted_4321 : PMIOPort  Port=2  Side=Left
  Redacted_2243 : PMIOPort  Port=3  Side=Left
  Redacted_707 : PMIOPort  Port=4  Side=Right
  Redacted_8636 : PMIOPort  Port=5  Side=Right

== system Electrical_System_2018b_obfs/Redacted_1221/Redacted_7996/Redacted_7418/Redacted_4377/Redacted_6082/Redacted_8502 ==
  Neutral_Negative : Subsystem  VariantControl=Variant1
  Positive_Neutral : Subsystem  VariantControl=Variant3
  Redacted_4068 : Subsystem  VariantControl=Variant2
  Redacted_389 : PMIOPort  Side=Left
  Redacted_6488 : PMIOPort  Port=2  Side=Left
  Redacted_5156 : PMIOPort  Port=3  Side=Left
  Redacted_180 : PMIOPort  Port=4  Side=Right
  Redacted_7018 : PMIOPort  Port=5  Side=Right
